simulink model "lindiscrmodel_lqi_uu"  (R2019a)
settings: Solver=VariableStepAuto  StartTime=0.0  StopTime=15  RelTol=1e-3
InitFcn:
  | lindiscrmodel
values from neighbouring files (symbols this model uses):
  K2_i = K2_lqi(1,5:6)    [lindiscrmodel.m]
  K2_lq = K2_lqi(1,1:4)    [lindiscrmodel.m]
  R_kal = cov(theta.data)    [lindiscrmodel.m]
  Ts = 0.01    [lindiscrmodel.m]
undefined symbols (not defined in the file or in its folder): DiscIntNeverNeededParam, Discrete, linmat, Time
libraries: ctrlSharedLib x1
settings Model: Creator=jessi  LastModifiedBy=jessi

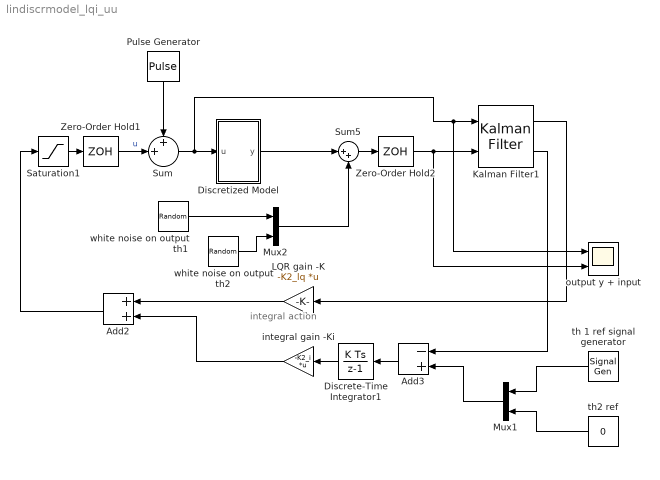
== system lindiscrmodel_lqi_uu ==
  note: integral action
  Add2 : Sum
  Add3 : Sum  Inputs=-+
  Discrete-Time Integrator1 : DiscreteIntegrator  SampleTime=Ts  ICPrevOutput=DiscIntNeverNeededParam  ICPrevScaledInput=DiscIntNeverNeededParam
  Discretized Model : Subsystem
  Kalman Filter1 : ctrlSharedLib/Kalman Filter  TimeDomain=Discrete-Time  UseCurrentEstimator=on  ModelSource=Individual A, B, C, D matrices  ModelSourceVariable=sysd2  A=linmat.A2  B=linmat.B2  C=linmat.C2  D=linmat.D2  NumberOfStates=1  NumberOfInputs=1  NumberOfOutputs=1  InitialEstimateSource=Dialog  X0=[0;0.05;0;0]  P0=10  UseK=off  UseGH=off  NumberOfProcessNoiseInputs=1  G=1  TimeInvariantG=on  H=0  TimeInvariantH=on  Q=0.000001*diag([1 1 1 1])  TimeInvariantQ=on  R=R_kal  TimeInvariantR=on  N=0  TimeInvariantN=on  AddInputPort=on  AddEnablePort=off  OutputEstimatedY=on  OutputP=off  Ts=Ts
      settings: SourceProductBaseCode=CT
  LQR gain -K : Gain  Gain=-K2_lq  Multiplication=Matrix(K*u)
  Mux1 : Mux  Inputs=2
  Mux2 : Mux  Inputs=2
  Pulse Generator : DiscretePulseGenerator  PulseType=Time based  Period=10  PulseWidth=5
  Saturation1 : Saturate  UpperLimit=1  LowerLimit=-1
  Sum : Sum  Inputs=++|
  Sum5 : Sum  Inputs=|++
  Zero-Order Hold1 : ZeroOrderHold  SampleTime=Ts
  Zero-Order Hold2 : ZeroOrderHold  SampleTime=Ts
  integral gain -Ki : Gain  Gain=-K2_i  Multiplication=Matrix(K*u)
  output y + input : Scope  NumInputPorts=2
  th 1 ref signal generator : SignalGenerator  Amplitude=0  Frequency=1/15
  th2 ref : Constant  Value=0  SampleTime=Ts
  white noise on output th1 : RandomNumber  Variance=1e-7  SampleTime=0.01
  white noise on output th2 : RandomNumber  Variance=1e-7  SampleTime=0.01
  wires:
  th2 ref/1 -> Mux1/2
  th 1 ref signal generator/1 -> Mux1/1
  white noise on output th1/1 -> Mux2/1
  white noise on output th2/1 -> Mux2/2
  Mux2/1 -> Sum5/2
  Sum5/1 -> Zero-Order Hold2/1
  Saturation1/1 -> Zero-Order Hold1/1
  Discretized Model/1(y) -> Sum5/1
  Kalman Filter1/1 -> LQR gain -K/1
  LQR gain -K/1 -> Add2/1
  Add2/1 -> Saturation1/1
  Kalman Filter1/2 -> Add3/1
  Mux1/1 -> Add3/2
  Discrete-Time Integrator1/1 -> integral gain -Ki/1
  Add3/1 -> Discrete-Time Integrator1/1
  integral gain -Ki/1 -> Add2/2
  Zero-Order Hold2/1 -> output y + input/2, Kalman Filter1/2
  Zero-Order Hold1/1 -> Sum/2  "u"
  Pulse Generator/1 -> Sum/1
  Sum/1 -> output y + input/1, Kalman Filter1/1, Discretized Model/1(u)

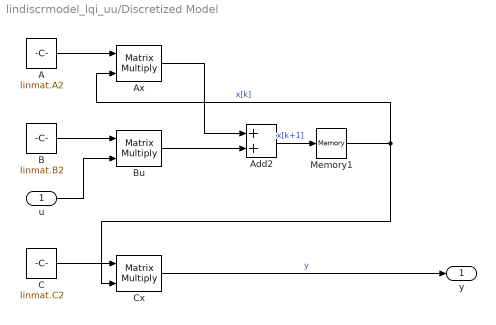
== system lindiscrmodel_lqi_uu/Discretized Model ==
  u : Inport
  A : Constant  Value=linmat.A2  SampleTime=Ts
  Add2 : Sum
  Ax : Product  Multiplication=Matrix(*)
  B : Constant  Value=linmat.B2  SampleTime=Ts
  Bu : Product  Multiplication=Matrix(*)
  C : Constant  Value=linmat.C2  SampleTime=Ts
  Cx : Product  Multiplication=Matrix(*)
  Memory1 : Memory  InitialCondition=[0;0.05;0;0]
  y : Outport
  wires:
  B/1 -> Bu/1
  Memory1/1 -> Cx/2, Ax/2  "x[k]"
  Add2/1 -> Memory1/1  "x[k+1]"
  C/1 -> Cx/1
  A/1 -> Ax/1
  u/1 -> Bu/2
  Ax/1 -> Add2/1
  Bu/1 -> Add2/2
  Cx/1 -> y/1  "y"
